simulink model "ElevatorAndMotor"  (R2023b)
settings: Solver=VariableStepAuto  StartTime=0.0  StopTime=10.0  RelTol=1e-3
settings Model: Creator=alalar1  LastModifiedBy=alalar1

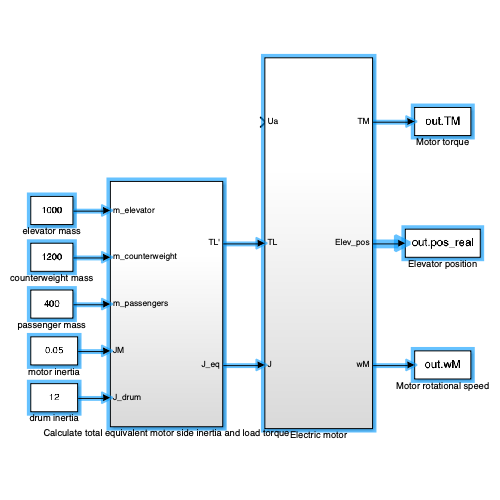
[thumbnail: Simulink's stored preview of the top-level diagram]
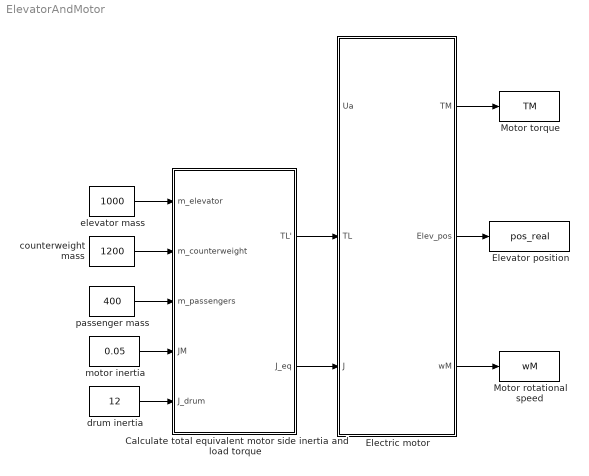
== system ElevatorAndMotor ==
  Calculate total equivalent motor side inertia and load torque : Subsystem
  Electric motor : Subsystem
  Elevator position : ToWorkspace  VariableName=pos_real  SaveFormat=Timeseries  SampleTime=-1
  Motor rotational speed : ToWorkspace  VariableName=wM  SaveFormat=Timeseries  SampleTime=-1
  Motor torque : ToWorkspace  VariableName=TM  SaveFormat=Timeseries  SampleTime=-1
  counterweight mass : Constant  Value=1200
  drum inertia : Constant  Value=12
  elevator mass : Constant  Value=1000
  motor inertia : Constant  Value=0.05
  passenger mass : Constant  Value=400
  wires:
  passenger mass/1 -> Calculate total equivalent motor side inertia and load torque/3(m_passengers)
  elevator mass/1 -> Calculate total equivalent motor side inertia and load torque/1(m_elevator)
  Electric motor/3(wM) -> Motor rotational speed/1
  Calculate total equivalent motor side inertia and load torque/1(TL') -> Electric motor/2(TL)
  drum inertia/1 -> Calculate total equivalent motor side inertia and load torque/5(J_drum)
  motor inertia/1 -> Calculate total equivalent motor side inertia and load torque/4(JM)
  counterweight mass/1 -> Calculate total equivalent motor side inertia and load torque/2(m_counterweight)
  Electric motor/1(TM) -> Motor torque/1
  Calculate total equivalent motor side inertia and load torque/2(J_eq) -> Electric motor/3(J)
  Electric motor/2(Elev_pos) -> Elevator position/1

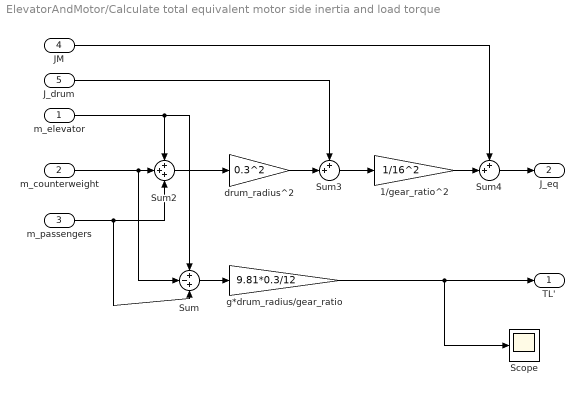
== system ElevatorAndMotor/Calculate total equivalent motor side inertia and load torque ==
  m_elevator : Inport
  m_counterweight : Inport  Port=2
  m_passengers : Inport  Port=3
  JM : Inport  Port=4
  J_drum : Inport  Port=5
  1/gear_ratio^2 : Gain  Gain=1/16^2
  Scope : Scope
  Sum : Sum  Inputs=+-+
  Sum2 : Sum  Inputs=+++
  Sum3 : Sum  Inputs=++|
  Sum4 : Sum  Inputs=++|
  drum_radius^2 : Gain  Gain=0.3^2
  g*drum_radius/gear_ratio : Gain  Gain=9.81*0.3/12
  TL' : Outport  VectorParamsAs1DForOutWhenUnconnected=off
  J_eq : Outport  Port=2  VectorParamsAs1DForOutWhenUnconnected=off
  wires:
  m_elevator/1 -> Sum/1, Sum2/1
  drum_radius^2/1 -> Sum3/2
  m_passengers/1 -> Sum2/3, Sum/3
  Sum2/1 -> drum_radius^2/1
  JM/1 -> Sum4/1
  J_drum/1 -> Sum3/1
  Sum3/1 -> 1/gear_ratio^2/1
  m_counterweight/1 -> Sum/2, Sum2/2
  1/gear_ratio^2/1 -> Sum4/2
  Sum4/1 -> J_eq/1
  Sum/1 -> g*drum_radius/gear_ratio/1
  g*drum_radius/gear_ratio/1 -> Scope/1, TL'/1

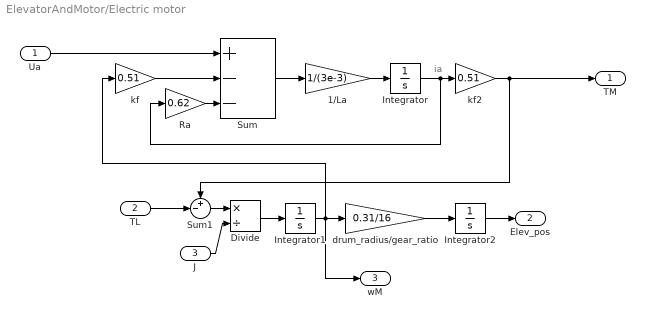
== system ElevatorAndMotor/Electric motor ==
  note: ia
  Ua : Inport
  TL : Inport  Port=2
  J : Inport  Port=3
  1/La : Gain  Gain=1/(3e-3)
  Divide : Product  Inputs=*/
  Integrator : Integrator
  Integrator1 : Integrator
  Integrator2 : Integrator
  Ra : Gain  Gain=0.62
  Sum : Sum  Inputs=+--
  Sum1 : Sum  Inputs=+-|
  drum_radius/gear_ratio : Gain  Gain=0.31/16
  kf : Gain  Gain=0.51
  kf2 : Gain  Gain=0.51
  TM : Outport  VectorParamsAs1DForOutWhenUnconnected=off
  Elev_pos : Outport  Port=2  VectorParamsAs1DForOutWhenUnconnected=off
  wM : Outport  Port=3  VectorParamsAs1DForOutWhenUnconnected=off
  wires:
  Integrator/1 -> Ra/1, kf2/1
  kf2/1 -> TM/1, Sum1/1
  1/La/1 -> Integrator/1
  Sum/1 -> 1/La/1
  Ua/1 -> Sum/1
  Ra/1 -> Sum/3
  kf/1 -> Sum/2
  Integrator1/1 -> wM/1, drum_radius/gear_ratio/1, kf/1
  Divide/1 -> Integrator1/1
  Sum1/1 -> Divide/1
  J/1 -> Divide/2
  TL/1 -> Sum1/2
  drum_radius/gear_ratio/1 -> Integrator2/1
  Integrator2/1 -> Elev_pos/1
